simulink model "pmsm_ajit"  (R2024a)
settings: Solver=FixedStepAuto  StartTime=0.0  StopTime=5  FixedStep=1e-3  RelTol=1e-3
libraries: simulink x6, spsControlledVoltageSourceLib x3, spsGroundLib x2, spsPermanentMagnetSynchronousMachineLib x2, spsThreePhaseSeriesRLCBranchLib x1, spsThreePhaseVIMeasurementLib x1, sps_lib x1
settings Model: Creator=ammarabdulrasheed  LastModifiedBy=ammarabdulrasheed

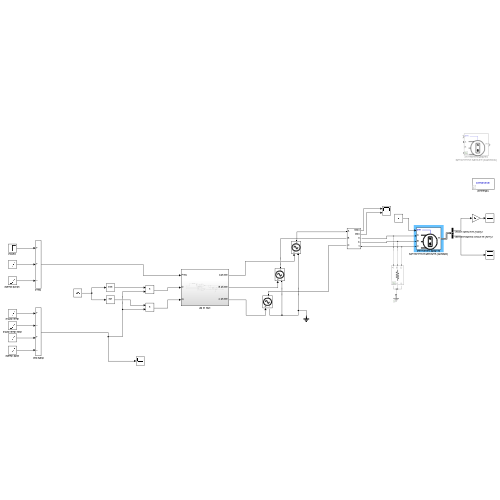
[thumbnail: Simulink's stored preview of the top-level diagram]
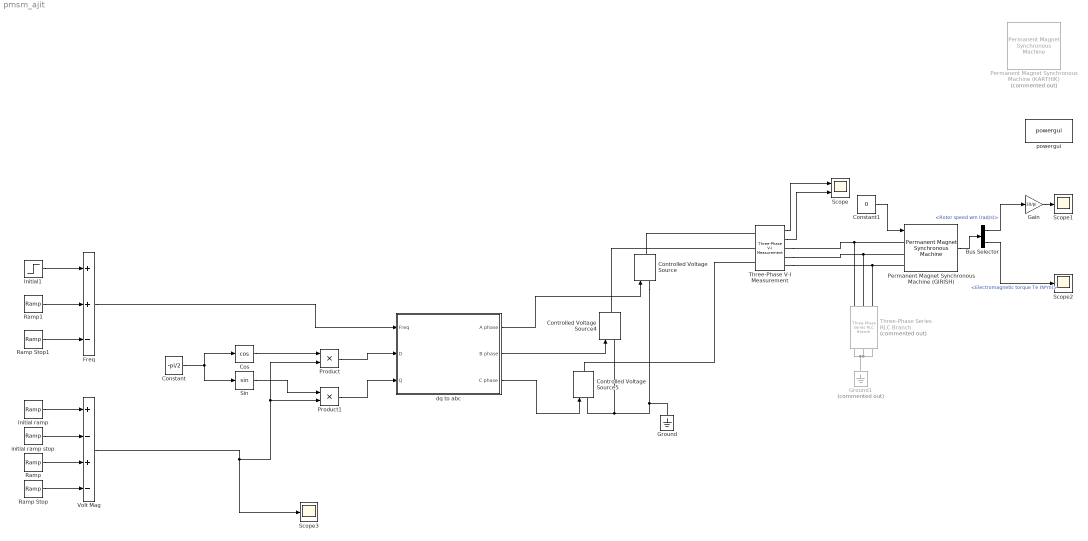
== system pmsm_ajit ==
  Bus Selector : BusSelector  OutputSignals=Rotor speed wm (rad/s),Electromagnetic torque Te (N*m)
  Constant : Constant  Value=-pi/2
  Constant1 : Constant  Value=0
  Controlled Voltage Source : spsControlledVoltageSourceLib/Controlled Voltage Source  Initialize=on  Source_Type=AC  Amplitude=0  Phase=0  Frequency=0  Measurements=None
  Controlled Voltage Source4 : spsControlledVoltageSourceLib/Controlled Voltage Source  Initialize=on  Source_Type=AC  Amplitude=0  Phase=0  Frequency=0  Measurements=None
  Controlled Voltage Source5 : spsControlledVoltageSourceLib/Controlled Voltage Source  Initialize=on  Source_Type=AC  Amplitude=0  Phase=0  Frequency=0  Measurements=None
  Cos : Trigonometry  Operator=cos
  Freq : Sum  Inputs=++-
  Gain : Gain  Gain=30/pi
  Ground : spsGroundLib/Ground  LConnTagsString=a
  Ground1 : spsGroundLib/Ground  Commented=on  LConnTagsString=a
  Initial ramp : simulink/Sources/Ramp  slope=20  start=0  InitialOutput=0
  Initial1 : Step  Time=0  After=0  SampleTime=0
  Permanent Magnet Synchronous Machine (GIRISH) : spsPermanentMagnetSynchronousMachineLib/Permanent Magnet Synchronous Machine  NbPhases=3  FluxDistribution=Sinusoidal  RotorType=Salient-pole  MechanicalLoad=Torque Tm  PresetModel=No  ShowDetailedParameters=on  MeasurementBus=off  Resistance=1.93  Inductance=8.5e-3  dqInductances=[45.56e-3,79.57e-3]  La=92.19e-3  MachineConstant=Flux linkage established by magnets (V.s)  Flux=0.311  VoltageCst=112.8183  TorqueCst=0.933  Flat=120  Mechanical=[0.003 0.001 2 0]  PolePairs=4  InitialConditions=[0,0, 0,0]  InitialConditions5ph=[0 0 0 0 0 0]  RefAngle=90 degrees behind phase A axis (modified Park)  IterativeDiscreteModel=Trapezoidal non iterative  TsBlock=-1  TsPowergui=0
  Permanent Magnet Synchronous Machine (KARTHIK) : spsPermanentMagnetSynchronousMachineLib/Permanent Magnet Synchronous Machine  Commented=on  NbPhases=3  FluxDistribution=Sinusoidal  RotorType=Round  MechanicalLoad=Torque Tm  PresetModel=No  ShowDetailedParameters=on  MeasurementBus=off  Resistance=1.15  Inductance=8.5e-3  dqInductances=[45.56e-3,79.57e-3]  La=24.3e-3  MachineConstant=Flux linkage established by magnets (V.s)  Flux=0.9426  VoltageCst=341.9375  TorqueCst=2.8278  Flat=120  Mechanical=[0.0145 0.00029 2 0]  PolePairs=4  InitialConditions=[0,0, 0,0]  InitialConditions5ph=[0 0 0 0 0 0]  RefAngle=90 degrees behind phase A axis (modified Park)  IterativeDiscreteModel=Trapezoidal non iterative  TsBlock=-1  TsPowergui=0
  Product : Product
  Product1 : Product
  Ramp : simulink/Sources/Ramp  slope=25*3.6  start=1 + 10/(3.6*25)  InitialOutput=0
  Ramp Stop : simulink/Sources/Ramp  slope=25*3.6  start=3  InitialOutput=0
  Ramp Stop1 : simulink/Sources/Ramp  slope=25  start=3  InitialOutput=0
  Ramp1 : simulink/Sources/Ramp  slope=25  start=1  InitialOutput=0
  Scope : Scope  NumInputPorts=2
  Scope1 : Scope
  Scope2 : Scope
  Scope3 : Scope
  Sin : Trigonometry
  Three-Phase Series RLC Branch : spsThreePhaseSeriesRLCBranchLib/Three-Phase Series RLC Branch  Commented=on  LConnTagsString=A|B|C  RConnTagsString=A|B|C  BranchType=R  Resistance=1e3  Inductance=1e-3  Capacitance=1e-6  Measurements=None
  Three-Phase V-I Measurement : spsThreePhaseVIMeasurementLib/Three-Phase V-I Measurement  VoltageMeasurement=phase-to-ground  SetLabelV=off  LabelV=Vabc  Vpu=off  VpuLL=off  CurrentMeasurement=yes  SetLabelI=off  LabelI=Iabc  Ipu=off  Pbase=100e6  Vbase=500e3  OutputType=Complex  PhasorSimulation=off  PSBequivalent=0
  Volt Mag : Sum  Inputs=+-+-
  dq to abc : Subsystem
  initial ramp stop : simulink/Sources/Ramp  slope=20  start=0.5  InitialOutput=0
  powergui : sps_lib/powergui  Priority=1  SimulationMode=Continuous  SampleTime=50e-6  frequency=60  Iterations=50  frequencyindice=0  Pbase=100e6  ErrMax=1e-4  UnitsV=kV  UnitsW=MW  buscounter=0  FunctionMessages=off  echomessages=off  EnableUseOfTLC=off  CurrentSourceSwitches=off  DisableSnubberDevices=off  DisableRonSwitches=off  DisableVfSwitches=off  DisplayEquations=off  AutomaticDiscreteSolvers=off  SolverType=Tustin/Backward Euler (TBE)  Interpol=off  ExternalGateDelay=off  methode=off  Ts=100  x0status=blocks  SPID=on  SwTol=0  HookPort=off  NonlinearTolerance=1e-4  nMaxIteration=100  ContinueOnMaxIteration=off  RestoreLinks=warning  ResistiveCurrentMeasurement=off  Frange=[0:2:500]  Ylog=off  Xlog=on  ShowGrid=off  save=off  variable=ZData  structure=0  ZoomFFT=off  StartTime=0.0  cycles=1  DisplayStyle=1  fundamental=60  FreqAxis=off  MaxFrequency=1000  frequencyindicesteady=1  RmsSteady=1  display=off
  wires:
  Ramp Stop1/1 -> Freq/3
  Initial1/1 -> Freq/1
  Ramp1/1 -> Freq/2
  Freq/1 -> dq to abc/1(Freq)
  Constant/1 -> Sin/1, Cos/1
  dq to abc/1(A phase) -> Controlled Voltage Source/1
  dq to abc/2(B phase) -> Controlled Voltage Source4/1
  dq to abc/3(C phase) -> Controlled Voltage Source5/1
  Three-Phase V-I Measurement/1 -> Scope/1
  Constant1/1 -> Permanent Magnet Synchronous Machine (GIRISH)/1
  Permanent Magnet Synchronous Machine (GIRISH)/1 -> Bus Selector/1
  Bus Selector/1 -> Gain/1  "<Rotor speed wm (rad/s)>"
  Cos/1 -> Product/1
  Product/1 -> dq to abc/2(D)
  Sin/1 -> Product1/1
  Product1/1 -> dq to abc/3(Q)
  Ramp Stop/1 -> Volt Mag/4
  Ramp/1 -> Volt Mag/3
  Initial ramp/1 -> Volt Mag/1
  initial ramp stop/1 -> Volt Mag/2
  Volt Mag/1 -> Scope3/1, Product1/2, Product/2
  Three-Phase V-I Measurement/2 -> Scope/2
  Bus Selector/2 -> Scope2/1  "<Electromagnetic torque Te (N*m)>"
  Gain/1 -> Scope1/1
  connections:
  Controlled Voltage Source/LConn1 -- Ground/LConn1 -- Controlled Voltage Source5/LConn1 -- Controlled Voltage Source4/LConn1
  Controlled Voltage Source/RConn1 -- Three-Phase V-I Measurement/LConn1
  Controlled Voltage Source4/RConn1 -- Three-Phase V-I Measurement/LConn2
  Controlled Voltage Source5/RConn1 -- Three-Phase V-I Measurement/LConn3
  Three-Phase V-I Measurement/RConn1 -- Permanent Magnet Synchronous Machine (GIRISH)/LConn1 -- Three-Phase Series RLC Branch/LConn1
  Three-Phase V-I Measurement/RConn2 -- Permanent Magnet Synchronous Machine (GIRISH)/LConn2 -- Three-Phase Series RLC Branch/LConn2
  Three-Phase V-I Measurement/RConn3 -- Permanent Magnet Synchronous Machine (GIRISH)/LConn3 -- Three-Phase Series RLC Branch/LConn3
  Three-Phase Series RLC Branch/RConn1 -- Three-Phase Series RLC Branch/RConn2 -- Three-Phase Series RLC Branch/RConn3 -- Ground1/LConn1

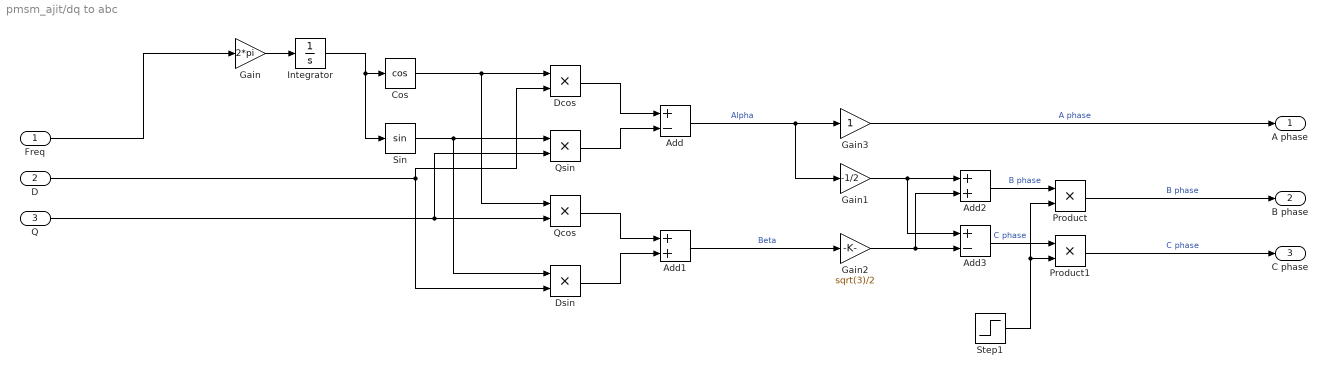
== system pmsm_ajit/dq to abc ==
  Freq : Inport
  D : Inport  Port=2
  Q : Inport  Port=3
  Add : Sum  Inputs=+-
  Add1 : Sum
  Add2 : Sum
  Add3 : Sum  Inputs=+-
  Cos : Trigonometry  Operator=cos
  Dcos : Product
  Dsin : Product
  Gain : Gain  Gain=2*pi
  Gain1 : Gain  Gain=-1/2
  Gain2 : Gain  Gain=sqrt(3)/2
  Gain3 : Gain
  Integrator : Integrator
  Product : Product
  Product1 : Product
  Qcos : Product
  Qsin : Product
  Sin : Trigonometry
  Step1 : Step  Time=0  SampleTime=0
  A phase : Outport
  B phase : Outport  Port=2
  C phase : Outport  Port=3
  wires:
  Product/1 -> B phase/1  "B phase"
  Add1/1 -> Gain2/1  "Beta"
  Product1/1 -> C phase/1  "C phase"
  D/1 -> Dsin/2, Dcos/2
  Dsin/1 -> Add1/2
  Freq/1 -> Gain/1
  Step1/1 -> Product1/2, Product/2
  Q/1 -> Qcos/2, Qsin/2
  Dcos/1 -> Add/1
  Gain/1 -> Integrator/1
  Gain3/1 -> A phase/1  "A phase"
  Cos/1 -> Qcos/1, Dcos/1
  Add2/1 -> Product/1  "B phase"
  Gain2/1 -> Add3/2, Add2/2
  Integrator/1 -> Sin/1, Cos/1
  Add3/1 -> Product1/1  "C phase"
  Sin/1 -> Dsin/1, Qsin/1
  Gain1/1 -> Add3/1, Add2/1
  Qsin/1 -> Add/2
  Qcos/1 -> Add1/1
  Add/1 -> Gain1/1, Gain3/1  "Alpha"
